simulink model "SimlinkModel_Observer"  (R2022b)
settings: Solver=VariableStepAuto  StartTime=0.0  StopTime=10  RelTol=1e-3
undefined symbols (not defined in the file): Aco, B, eqmatrix, K, Ke, Ki
settings Model: Creator=Abdelateef  LastModifiedBy=عالم الكمبيوتر

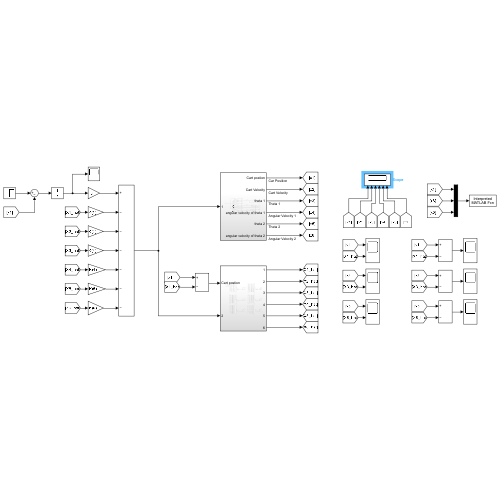
[thumbnail: Simulink's stored preview of the top-level diagram]
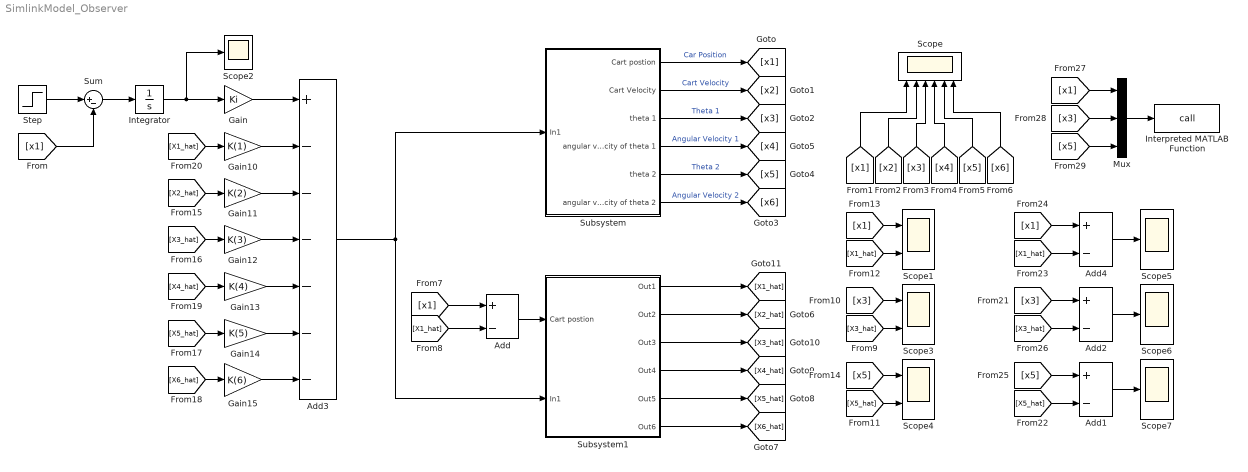
== system SimlinkModel_Observer ==
  Add{,1..2,4} (4 alike) : Sum  Inputs=+-
  Add3 : Sum  Inputs=+------
  Gain : Gain  Gain=Ki
  Gain10 : Gain  Gain=K(1)
  Gain11 : Gain  Gain=K(2)
  Gain12 : Gain  Gain=K(3)
  Gain13 : Gain  Gain=K(4)
  Gain14 : Gain  Gain=K(5)
  Gain15 : Gain  Gain=K(6)
  Integrator : Integrator
  Interpreted MATLAB Function : MATLABFcn  MATLABFcn=call  OutputDimensions=0
  Mux : Mux  Inputs=3
  Scope : Scope  NumInputPorts=6
  Scope1 : Scope  NumInputPorts=2
  Scope{2,5..7} (4 alike) : Scope
  Scope3 : Scope  NumInputPorts=2
  Scope4 : Scope  NumInputPorts=2
  Step : Step  Time=0  SampleTime=0
  Subsystem : Subsystem
  Subsystem1 : Subsystem
  Sum : Sum  Inputs=|+-
  wires:
  Gain10/1 -> Add3/2
  Gain11/1 -> Add3/3
  Gain12/1 -> Add3/4
  Gain13/1 -> Add3/5
  Gain14/1 -> Add3/6
  Gain15/1 -> Add3/7
  Gain/1 -> Add3/1
  Integrator/1 -> Scope2/1, Gain/1
  Sum/1 -> Integrator/1
  [x1] -> Sum/2
  Subsystem/1(Cart postion) -> [x1]  "Car Position"
  Subsystem/2(Cart Velocity) -> [x2]  "Cart Velocity"
  Subsystem/3(theta 1) -> [x3]  "Theta 1"
  Subsystem/4(angular velocity of theta 1) -> [x4]  "Angular Velocity 1"
  Subsystem/5(theta 2) -> [x5]  "Theta 2"
  Subsystem/6(angular velocity of theta 2) -> [x6]  "Angular Velocity 2"
  Add3/1 -> Subsystem/1(In1), Subsystem1/2(In1)
  [x1] -> Add/1
  [X1_hat] -> Add/2
  [X5_hat] -> Gain14/1
  [X2_hat] -> Gain11/1
  [X4_hat] -> Gain13/1
  [X3_hat] -> Gain12/1
  [X6_hat] -> Gain15/1
  [X1_hat] -> Gain10/1
  Add/1 -> Subsystem1/1(Cart postion)
  Subsystem1/1(Out1) -> [X1_hat]
  Subsystem1/2(Out2) -> [X2_hat]
  Subsystem1/3(Out3) -> [X3_hat]
  Subsystem1/4(Out4) -> [X4_hat]
  Subsystem1/5(Out5) -> [X5_hat]
  Subsystem1/6(Out6) -> [X6_hat]
  [x1] -> Scope/1
  [x2] -> Scope/2
  [x3] -> Scope/3
  [x4] -> Scope/4
  [x5] -> Scope/5
  [x6] -> Scope/6
  [x1] -> Scope1/1
  [X1_hat] -> Scope1/2
  Step/1 -> Sum/1
  [x3] -> Scope3/1
  [X3_hat] -> Scope3/2
  [x5] -> Scope4/1
  [X5_hat] -> Scope4/2
  [X1_hat] -> Add4/2
  [x1] -> Add4/1
  [x3] -> Add2/1
  [X3_hat] -> Add2/2
  [x5] -> Add1/1
  [X5_hat] -> Add1/2
  Add4/1 -> Scope5/1
  Add2/1 -> Scope6/1
  Add1/1 -> Scope7/1
  Mux/1 -> Interpreted MATLAB Function/1
  [x1] -> Mux/1
  [x3] -> Mux/2
  [x5] -> Mux/3

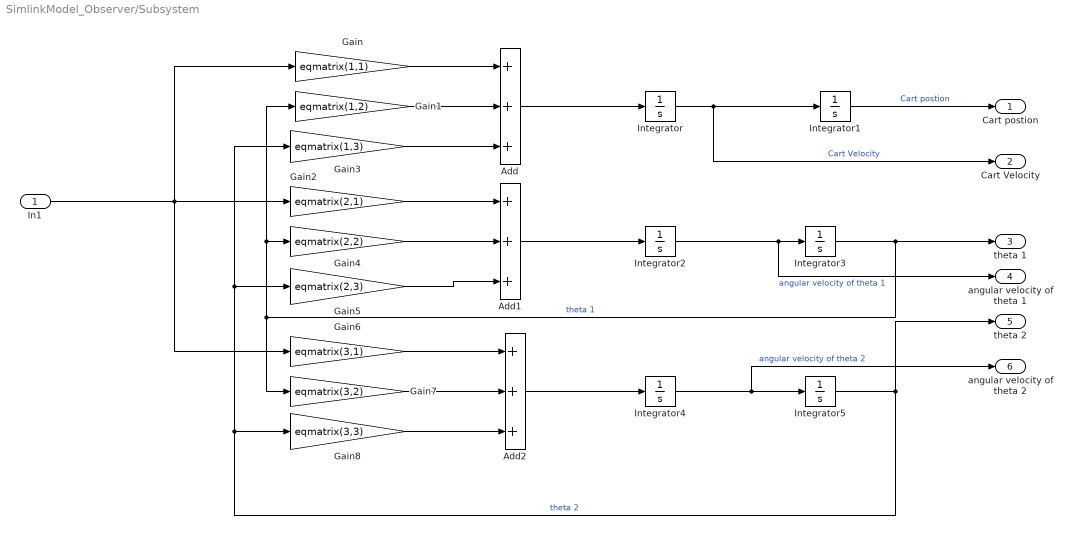
== system SimlinkModel_Observer/Subsystem ==
  In1 : Inport
  Add : Sum  Inputs=+++
  Add1 : Sum  Inputs=+++
  Add2 : Sum  Inputs=+++
  Gain : Gain  Gain=eqmatrix(1,1)
  Gain1 : Gain  Gain=eqmatrix(1,2)
  Gain2 : Gain  Gain=eqmatrix(2,1)
  Gain3 : Gain  Gain=eqmatrix(1,3)
  Gain4 : Gain  Gain=eqmatrix(2,2)
  Gain5 : Gain  Gain=eqmatrix(2,3)
  Gain6 : Gain  Gain=eqmatrix(3,1)
  Gain7 : Gain  Gain=eqmatrix(3,2)
  Gain8 : Gain  Gain=eqmatrix(3,3)
  Integrator{,1..5} (6 alike) : Integrator
  Cart postion : Outport
  Cart Velocity : Outport  Port=2
  theta 1 : Outport  Port=3
  angular velocity of theta 1 : Outport  Port=4
  theta 2 : Outport  Port=5
  angular velocity of theta 2 : Outport  Port=6
  wires:
  Gain2/1 -> Add1/1
  Gain4/1 -> Add1/2
  Integrator5/1 -> theta 2/1, Gain3/1, Gain5/1, Gain8/1  "theta 2"
  Integrator1/1 -> Cart postion/1  "Cart postion"
  Gain8/1 -> Add2/3
  Gain7/1 -> Add2/2
  Integrator4/1 -> angular velocity of theta 2/1, Integrator5/1  "angular velocity of theta 2"
  Integrator/1 -> Cart Velocity/1, Integrator1/1  "Cart Velocity"
  Integrator3/1 -> Gain1/1, Gain4/1, Gain7/1, theta 1/1  "theta 1"
  In1/1 -> Gain6/1, Gain2/1, Gain/1
  Gain1/1 -> Add/2
  Add/1 -> Integrator/1
  Gain3/1 -> Add/3
  Gain6/1 -> Add2/1
  Gain5/1 -> Add1/3
  Add2/1 -> Integrator4/1
  Integrator2/1 -> angular velocity of theta 1/1, Integrator3/1  "angular velocity of theta 1"
  Gain/1 -> Add/1
  Add1/1 -> Integrator2/1

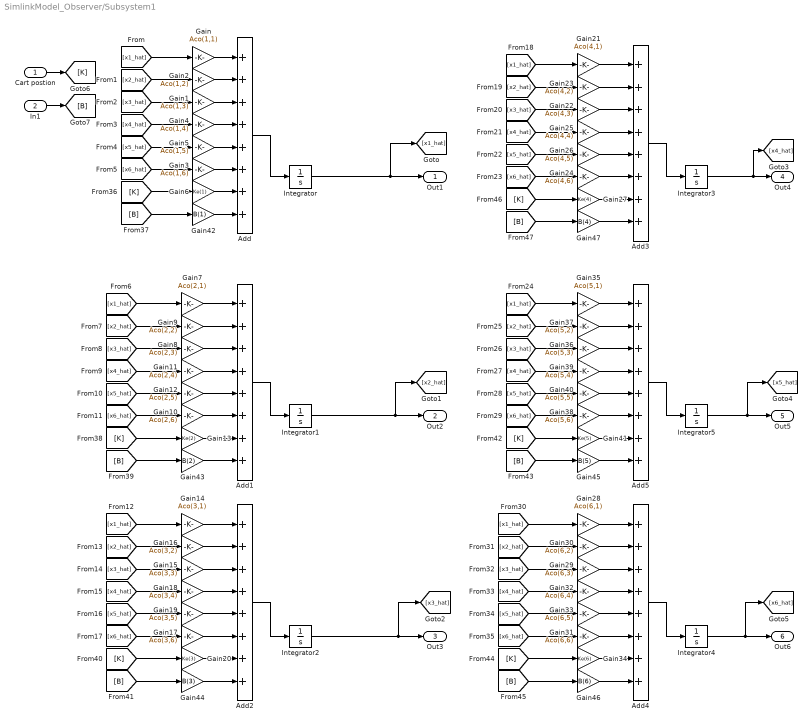
== system SimlinkModel_Observer/Subsystem1 ==
  Cart postion : Inport
  In1 : Inport  Port=2
  Add{,1..5} (6 alike) : Sum  Inputs=++++++++
  Gain : Gain  Gain=Aco(1,1)
  Gain1 : Gain  Gain=Aco(1,3)
  Gain10 : Gain  Gain=Aco(2,6)
  Gain11 : Gain  Gain=Aco(2,4)
  Gain12 : Gain  Gain=Aco(2,5)
  Gain13 : Gain  Gain=Ke(2)
  Gain14 : Gain  Gain=Aco(3,1)
  Gain15 : Gain  Gain=Aco(3,3)
  Gain16 : Gain  Gain=Aco(3,2)
  Gain17 : Gain  Gain=Aco(3,6)
  Gain18 : Gain  Gain=Aco(3,4)
  Gain19 : Gain  Gain=Aco(3,5)
  Gain2 : Gain  Gain=Aco(1,2)
  Gain20 : Gain  Gain=Ke(3)
  Gain21 : Gain  Gain=Aco(4,1)
  Gain22 : Gain  Gain=Aco(4,3)
  Gain23 : Gain  Gain=Aco(4,2)
  Gain24 : Gain  Gain=Aco(4,6)
  Gain25 : Gain  Gain=Aco(4,4)
  Gain26 : Gain  Gain=Aco(4,5)
  Gain27 : Gain  Gain=Ke(4)
  Gain28 : Gain  Gain=Aco(6,1)
  Gain29 : Gain  Gain=Aco(6,3)
  Gain3 : Gain  Gain=Aco(1,6)
  Gain30 : Gain  Gain=Aco(6,2)
  Gain31 : Gain  Gain=Aco(6,6)
  Gain32 : Gain  Gain=Aco(6,4)
  Gain33 : Gain  Gain=Aco(6,5)
  Gain34 : Gain  Gain=Ke(6)
  Gain35 : Gain  Gain=Aco(5,1)
  Gain36 : Gain  Gain=Aco(5,3)
  Gain37 : Gain  Gain=Aco(5,2)
  Gain38 : Gain  Gain=Aco(5,6)
  Gain39 : Gain  Gain=Aco(5,4)
  Gain4 : Gain  Gain=Aco(1,4)
  Gain40 : Gain  Gain=Aco(5,5)
  Gain41 : Gain  Gain=Ke(5)
  Gain42 : Gain  Gain=B(1)
  Gain43 : Gain  Gain=B(2)
  Gain44 : Gain  Gain=B(3)
  Gain45 : Gain  Gain=B(5)
  Gain46 : Gain  Gain=B(6)
  Gain47 : Gain  Gain=B(4)
  Gain5 : Gain  Gain=Aco(1,5)
  Gain6 : Gain  Gain=Ke(1)
  Gain7 : Gain  Gain=Aco(2,1)
  Gain8 : Gain  Gain=Aco(2,3)
  Gain9 : Gain  Gain=Aco(2,2)
  Integrator : Integrator  InitialCondition=-0.001
  Integrator1 : Integrator
  Integrator2 : Integrator  InitialCondition=0.079
  Integrator3 : Integrator
  Integrator4 : Integrator
  Integrator5 : Integrator  InitialCondition=0.079
  Out1 : Outport
  Out2 : Outport  Port=2
  Out3 : Outport  Port=3
  Out4 : Outport  Port=4
  Out5 : Outport  Port=5
  Out6 : Outport  Port=6
  wires:
  Add/1 -> Integrator/1
  Gain/1 -> Add/1
  Gain2/1 -> Add/2
  Gain1/1 -> Add/3
  Integrator/1 -> [x1_hat], Out1/1
  Gain4/1 -> Add/4
  Gain3/1 -> Add/6
  Gain5/1 -> Add/5
  Gain11/1 -> Add1/4
  Add1/1 -> Integrator1/1
  Gain9/1 -> Add1/2
  Gain7/1 -> Add1/1
  Gain13/1 -> Add1/7
  Gain10/1 -> Add1/6
  Gain8/1 -> Add1/3
  Gain12/1 -> Add1/5
  Gain18/1 -> Add2/4
  Add2/1 -> Integrator2/1
  Gain16/1 -> Add2/2
  Gain14/1 -> Add2/1
  Gain20/1 -> Add2/7
  Gain17/1 -> Add2/6
  Gain15/1 -> Add2/3
  Gain19/1 -> Add2/5
  Integrator2/1 -> [x3_hat], Out3/1
  Gain25/1 -> Add3/4
  Add3/1 -> Integrator3/1
  Gain23/1 -> Add3/2
  Gain21/1 -> Add3/1
  Gain27/1 -> Add3/7
  Gain24/1 -> Add3/6
  Gain22/1 -> Add3/3
  Gain26/1 -> Add3/5
  Gain39/1 -> Add5/4
  Add5/1 -> Integrator5/1
  Gain37/1 -> Add5/2
  Gain35/1 -> Add5/1
  Gain41/1 -> Add5/7
  Gain38/1 -> Add5/6
  Gain36/1 -> Add5/3
  Gain40/1 -> Add5/5
  Gain32/1 -> Add4/4
  Add4/1 -> Integrator4/1
  Gain30/1 -> Add4/2
  Gain28/1 -> Add4/1
  Gain34/1 -> Add4/7
  Gain31/1 -> Add4/6
  Gain29/1 -> Add4/3
  Gain33/1 -> Add4/5
  Integrator3/1 -> [x4_hat], Out4/1
  Integrator5/1 -> [x5_hat], Out5/1
  Integrator4/1 -> [x6_hat], Out6/1
  Gain6/1 -> Add/7
  Gain42/1 -> Add/8
  [x1_hat] -> Gain/1
  Integrator1/1 -> [x2_hat], Out2/1
  [x2_hat] -> Gain2/1
  [x3_hat] -> Gain1/1
  [x4_hat] -> Gain4/1
  [x5_hat] -> Gain5/1
  [x6_hat] -> Gain3/1
  [x1_hat] -> Gain7/1
  [x3_hat] -> Gain8/1
  [x2_hat] -> Gain9/1
  [x6_hat] -> Gain10/1
  [x5_hat] -> Gain12/1
  [x4_hat] -> Gain11/1
  [x1_hat] -> Gain14/1
  [x3_hat] -> Gain15/1
  [x2_hat] -> Gain16/1
  [x6_hat] -> Gain17/1
  [x5_hat] -> Gain19/1
  [x4_hat] -> Gain18/1
  [x1_hat] -> Gain21/1
  [x3_hat] -> Gain22/1
  [x2_hat] -> Gain23/1
  [x6_hat] -> Gain24/1
  [x5_hat] -> Gain26/1
  [x4_hat] -> Gain25/1
  [x1_hat] -> Gain35/1
  [x3_hat] -> Gain36/1
  [x2_hat] -> Gain37/1
  [x6_hat] -> Gain38/1
  [x5_hat] -> Gain40/1
  [x4_hat] -> Gain39/1
  [x1_hat] -> Gain28/1
  [x3_hat] -> Gain29/1
  [x2_hat] -> Gain30/1
  [x6_hat] -> Gain31/1
  [x5_hat] -> Gain33/1
  [x4_hat] -> Gain32/1
  Cart postion/1 -> [K]
  In1/1 -> [B]
  [K] -> Gain6/1
  [B] -> Gain42/1
  Gain43/1 -> Add1/8
  [K] -> Gain13/1
  [B] -> Gain43/1
  [K] -> Gain20/1
  [B] -> Gain44/1
  Gain44/1 -> Add2/8
  Gain45/1 -> Add5/8
  [B] -> Gain45/1
  [K] -> Gain41/1
  Gain46/1 -> Add4/8
  [K] -> Gain34/1
  [B] -> Gain46/1
  [K] -> Gain27/1
  [B] -> Gain47/1
  Gain47/1 -> Add3/8
